simulink model "PIZANO_LAB5_part1_2"  (Simulink 10.0)
settings: Solver=FixedStepAuto  StartTime=0.0  StopTime=6  FixedStep=0.001  RelTol=1e-3
libraries: simulink_extras x2, simulink x1
settings Model: Creator=XxaemaeThxX  LastModifiedBy=XxaemaeThxX
settings DataIOCC: SaveFormat=Dataset  ReturnWorkspaceOutputs=on
settings OptimizationCC: LifeSpan=auto
settings DebuggingCC: UnderspecifiedInitializationDetection=Simplified  MergeDetectMultiDrivingBlocksExec=error  SFUnexpectedBacktrackingDiag=error  SFNoUnconditionalDefaultTransitionDiag=error  SFExecutionAtInitializationDiag=warning  ArithmeticOperatorsInVariantConditions=error
settings HardwareCC: ProdBitPerPointer=64  ProdBitPerSizeT=64  ProdBitPerPtrDiffT=64  ProdLargestAtomicFloat=Float  ProdIntDivRoundTo=Zero  ProdEndianess=LittleEndian  ProdWordSize=64  ProdHWDeviceType=Intel->x86-64 (Windows64)
settings ModelReferenceCC: PropagateSignalLabelsOutOfModel=on
settings SFSimCC: SimUseLocalCustomCode=on  CustomCodeUndefinedFunction=FilterOut
settings RTWCC: RTWUseLocalCustomCode=on
settings CodeAppCC: StateflowObjectComments=off
settings GRTTargetCC: TargetLangStandard=C99 (ISO)  CombineOutputUpdateFcns=on  GRTInterface=off
settings ConfigComp: CovMetricSettings=dwe  CovHtmlReporting=off  CovSaveCumulativeToWorkspaceVar=off  CovSaveSingleToWorkspaceVar=off

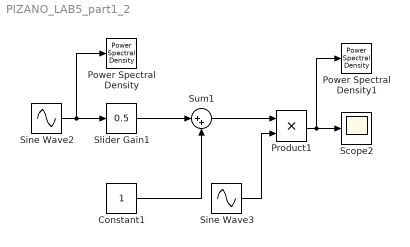
== system PIZANO_LAB5_part1_2 ==
  Constant1 : Constant
  Power Spectral Density : simulink_extras/Additional Sinks/Power Spectral Density  npts=512  fftpts=4096  HowOften=64  sampleT=0.001
      settings: SourceProductName=Simulink  SourceProductBaseCode=SL
  Power Spectral Density1 : simulink_extras/Additional Sinks/Power Spectral Density  npts=512  fftpts=4096  HowOften=64  sampleT=0.001
      settings: SourceProductName=Simulink  SourceProductBaseCode=SL
  Product1 : Product  RndMeth=Zero
  Scope2 : Scope
  Sine Wave2 : Sin  Frequency=5  SampleTime=0
  Sine Wave3 : Sin  Amplitude=2  Frequency=200  SampleTime=0
  Slider Gain1 : simulink/Math Operations/Slider Gain  gain=0.5  low=0  high=2
  Sum1 : Sum  Inputs=|++
  wires:
  Sine Wave3/1 -> Product1/2
  Slider Gain1/1 -> Sum1/1
  Sine Wave2/1 -> Slider Gain1/1, Power Spectral Density/1
  Product1/1 -> Scope2/1, Power Spectral Density1/1
  Constant1/1 -> Sum1/2
  Sum1/1 -> Product1/1
